simulink model "Lab5_Ris_2_16"  (Simulink 10.2)
settings: Solver=VariableStepAuto  StartTime=0.0  StopTime=0.128  RelTol=1e-3
libraries: commrandsrc3 x2, commseqgen3 x1
settings Model: Creator=Newtr  LastModifiedBy=Newtr
settings DataIOCC: SaveFormat=Dataset  SignalLoggingSaveFormat=Dataset  ReturnWorkspaceOutputs=on
settings OptimizationCC: LifeSpan=auto
settings DebuggingCC: UnderspecifiedInitializationDetection=Simplified  MergeDetectMultiDrivingBlocksExec=error  FcnCallInpInsideContextMsg=error  SFUnexpectedBacktrackingDiag=error  SFNoUnconditionalDefaultTransitionDiag=error  SFExecutionAtInitializationDiag=warning  ArithmeticOperatorsInVariantConditions=error
settings HardwareCC: ProdBitPerPointer=64  ProdBitPerSizeT=64  ProdBitPerPtrDiffT=64  ProdLargestAtomicFloat=Float  ProdIntDivRoundTo=Zero  ProdEndianess=LittleEndian  ProdWordSize=64  ProdHWDeviceType=Intel->x86-64 (Windows64)
settings ModelReferenceCC: PropagateSignalLabelsOutOfModel=on
settings SFSimCC: SimUseLocalCustomCode=on  CustomCodeUndefinedFunction=FilterOut
settings RTWCC: RTWUseLocalCustomCode=on
settings CodeAppCC: StateflowObjectComments=off
settings GRTTargetCC: TargetLangStandard=C99 (ISO)  CombineOutputUpdateFcns=on  GRTInterface=off
settings ConfigComp: CovMetricSettings=dwe  CovSaveCumulativeToWorkspaceVar=off  CovSaveSingleToWorkspaceVar=off  CovExternalEMLEnable=on

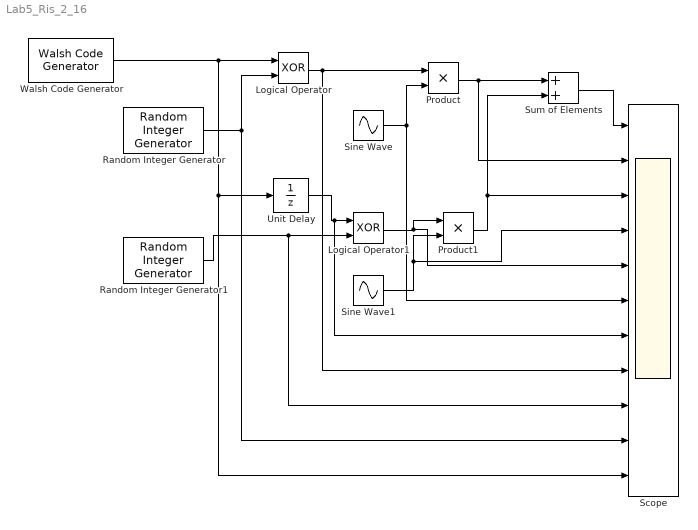
== system Lab5_Ris_2_16 ==
  Logical Operator : Logic  Operator=XOR  AllPortsSameDT=off  OutDataTypeStr=boolean
  Logical Operator1 : Logic  Operator=XOR  AllPortsSameDT=off  OutDataTypeStr=boolean
  Product : Product
  Product1 : Product
  Random Integer Generator : commrandsrc3/Random Integer Generator  SetSize=2  SeedSource=Parameter  Seed=12786  SampleTime=1/1.2288/10^6  SamplesPerFrame=1  OutputDataType=double  SimulateUsing=Interpreted execution
  Random Integer Generator1 : commrandsrc3/Random Integer Generator  SetSize=2  SeedSource=Parameter  Seed=01675  SampleTime=1/1.2288/10^6  SamplesPerFrame=1  OutputDataType=double  SimulateUsing=Interpreted execution
  Scope : Scope  NumInputPorts=11
  Sine Wave : Sin  SampleTime=0
  Sine Wave1 : Sin  SampleTime=0
  Sum of Elements : Sum
  Unit Delay : UnitDelay  SampleTime=-1  HasFrameUpgradeWarning=on
  Walsh Code Generator : commseqgen3/Walsh Code Generator  Length=128  Index=86  SampleTime=1/1.2288/10^6  SamplesPerFrame=1  OutputDataType=double  SimulateUsing=Code generation
      settings: SourceProductBaseCode=CM
  wires:
  Walsh Code Generator/1 -> Unit Delay/1, Scope/11, Logical Operator/1
  Random Integer Generator/1 -> Scope/10, Logical Operator/2
  Random Integer Generator1/1 -> Logical Operator1/2, Scope/9
  Unit Delay/1 -> Scope/7, Logical Operator1/1
  Logical Operator/1 -> Scope/8, Product/1
  Sine Wave/1 -> Scope/6, Product/2
  Sine Wave1/1 -> Scope/4, Product1/2
  Logical Operator1/1 -> Scope/5, Product1/1
  Product1/1 -> Scope/3, Sum of Elements/2
  Product/1 -> Scope/2, Sum of Elements/1
  Sum of Elements/1 -> Scope/1
